simulink model "Tema_bonus_Pisai_Daria_PC5_1"  (R2024b)
settings: Solver=FixedStepAuto  StartTime=0.0  StopTime=1500  FixedStep=0.01  RelTol=1e-3
model workspace (MAT data in the model file):
  a0 = 0.32
  a1 = 435
  a2 = 75000
  b1 = 0.32
  b21 = 300
  b22 = 0.3
  c1 = 0.2
settings Model: Creator=dariapisai  LastModifiedBy=dariapisai

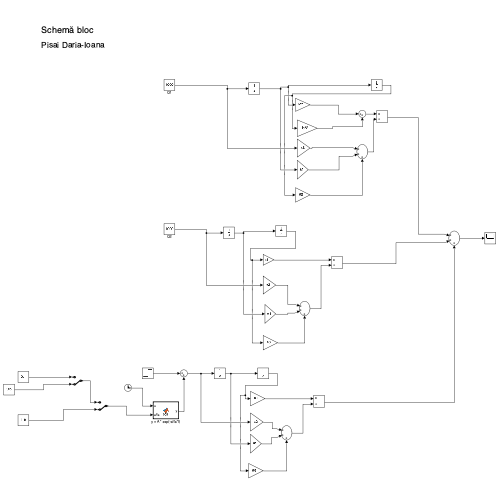
[thumbnail: Simulink's stored preview of the top-level diagram]
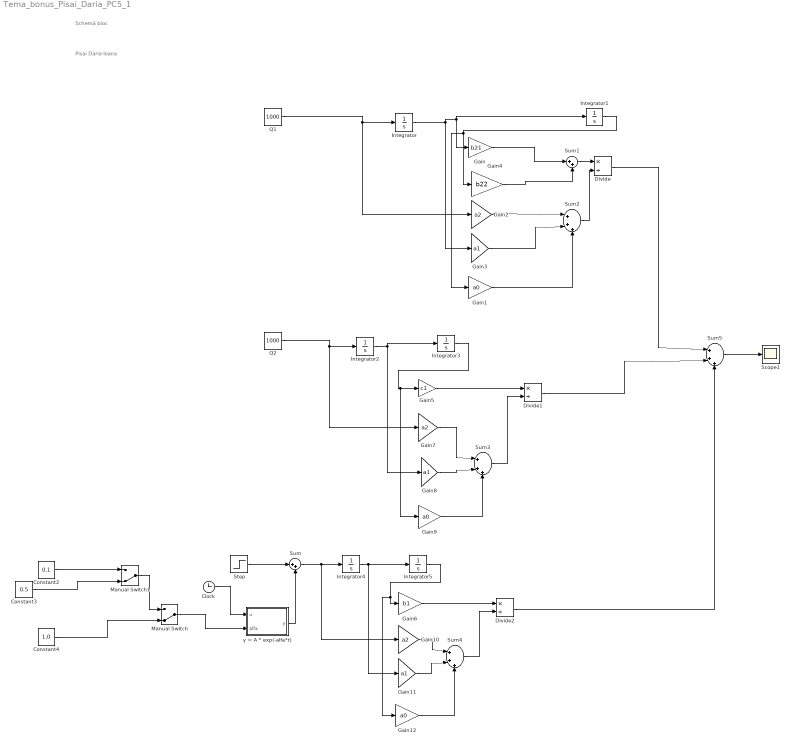
== system Tema_bonus_Pisai_Daria_PC5_1 ==
  note: Pisai Daria-Ioana
  note: Schemă bloc
  Clock : Clock
      settings: Decimation=1000
  Constant2 : Constant  Value=0.1
  Constant3 : Constant  Value=0.5
  Constant4 : Constant  Value=1.0
  Divide : Product  Inputs=*/
  Divide1 : Product  Inputs=*/
  Divide2 : Product  Inputs=*/
  Gain : Gain  Gain=b21
  Gain1 : Gain  Gain=a0
  Gain10 : Gain  Gain=a2
  Gain11 : Gain  Gain=a1
  Gain12 : Gain  Gain=a0
  Gain2 : Gain  Gain=a2
  Gain3 : Gain  Gain=a1
  Gain4 : Gain  Gain=b22
  Gain5 : Gain  Gain=c1
  Gain6 : Gain  Gain=b1
  Gain7 : Gain  Gain=a2
  Gain8 : Gain  Gain=a1
  Gain9 : Gain  Gain=a0
  Integrator{,1..5} (6 alike) : Integrator
  Manual Switch : ManualSwitch  CurrentSetting=0
  Manual Switch1 : ManualSwitch  CurrentSetting=0
  Q1 : Constant  Value=1000
  Q2 : Constant  Value=1000
  Scope1 : Scope
  Step : Step  Time=5  SampleTime=0
  Sum : Sum  Inputs=|++
  Sum1 : Sum  Inputs=|++
  Sum{2..5} (4 alike) : Sum  Inputs=|+++
  y = A * exp(-alfa*t) : MATLAB Function  TreatAsAtomicUnit=on
  wires:
  Step/1 -> Sum/1
  y = A * exp(-alfa*t)/1(y) -> Sum/2
  Sum/1 -> Gain10/1, Integrator4/1
  Integrator/1 -> Gain/1, Integrator1/1, Gain3/1
  Integrator1/1 -> Gain4/1, Gain1/1
  Gain/1 -> Sum1/1
  Gain4/1 -> Sum1/2
  Sum1/1 -> Divide/1
  Q1/1 -> Gain2/1, Integrator/1
  Gain2/1 -> Sum2/1
  Gain3/1 -> Sum2/2
  Gain1/1 -> Sum2/3
  Sum2/1 -> Divide/2
  Q2/1 -> Gain7/1, Integrator2/1
  Integrator2/1 -> Integrator3/1, Gain8/1
  Gain5/1 -> Divide1/1
  Gain7/1 -> Sum3/1
  Gain8/1 -> Sum3/2
  Integrator3/1 -> Gain9/1, Gain5/1
  Gain9/1 -> Sum3/3
  Sum3/1 -> Divide1/2
  Constant2/1 -> Manual Switch1/1
  Constant3/1 -> Manual Switch1/2
  Constant4/1 -> Manual Switch/2
  Manual Switch/1 -> y = A * exp(-alfa*t)/2(alfa)
  Clock/1 -> y = A * exp(-alfa*t)/1(u)
  Integrator4/1 -> Gain11/1, Integrator5/1
  Integrator5/1 -> Gain12/1, Gain6/1
  Gain6/1 -> Divide2/1
  Gain10/1 -> Sum4/1
  Gain12/1 -> Sum4/3
  Gain11/1 -> Sum4/2
  Sum4/1 -> Divide2/2
  Divide/1 -> Sum5/1
  Divide1/1 -> Sum5/2
  Divide2/1 -> Sum5/3
  Sum5/1 -> Scope1/1
  Manual Switch1/1 -> Manual Switch/1

== matlab function Tema_bonus_Pisai_Daria_PC5_1/y = A * exp(-alfa*t) ==
  data: u input; y output; alfa input
function y = fcn(u, alfa)

A = 2;

y = A*exp((-alfa)*u);

end
